simulink model "simulation2_Fault"  (R2018a)
settings: Solver=FixedStepAuto  StartTime=0.0  StopTime=2000  FixedStep=0.1  RelTol=1e-3
values from neighbouring files (symbols this model uses):
  C_wn = C_w(:,4)    [Sim1.m]    (also in Sim3.m; Sim4_EKF.m; Sim4_Nolinear.m; Sim5_Nolinear.m)
  C_wx = C_w(:,2)    [Sim1.m]    (also in Sim3.m; Sim4_EKF.m; Sim4_Nolinear.m; Sim5_Nolinear.m)
  C_wy = C_w(:,3)    [Sim1.m]    (also in Sim3.m; Sim4_EKF.m; Sim4_Nolinear.m; Sim5_Nolinear.m)
  Ce = inv(W)*Be'/(Be/W*Be')    [Sim2.m]    (also in Sim3.m; Sim4_EKF.m; Sim4_Nolinear.m; Sim5_Nolinear.m)
  getPos = [0;0;1]    [Sim2.m]    (also in Sim3.m; Sim4_EKF.m; Sim4_Nolinear.m; Sim5_Nolinear.m)
  getVel = [0;1;0]    [Sim2.m]    (also in Sim3.m; Sim4_EKF.m; Sim4_Nolinear.m; Sim5_Nolinear.m)
  h = 0.1    [Sim1.m]    (also in Sim2.m; Sim3.m; Sim4_EKF.m; Sim4_Nolinear.m)
  Kd = 7*[2*M3(1)*Omega 0 0; 0 3*M3(2,2)*Omega 0; 0 0 20*M(3,3)*Omega]    [Sim2.m]    (also in Sim3.m; Sim4_EKF.m; Sim4_Nolinear.m; Sim5_Nolinear.m = 7*[30*M3(1)*Omega 0 0; 0 150*M3(2,2)*Omega 0; 0 0 30*M(3,3)*)
  Ki = 100*(omega/10)*[M3(1)*omega^2 0 0;0 0.05*M3(2,2)*omega^2 0; 0 0 M3(3,3)*omega^2 ]*2    [Sim2.m]    (also in Sim3.m; Sim4_EKF.m; Sim4_Nolinear.m; Sim5_Nolinear.m = 10*(omega/10)*[30*M3(1)*omega^2 0 0;0 150*M3(2,2)*omega^2 0;)
  Kp = 50*[6*M3(1)*omega^2 0 0;0 M3(2,2)*omega^2 0; 0 0 10*M3(3,3)*omega^2 ]    [Sim2.m]    (also in Sim3.m; Sim4_EKF.m; Sim4_Nolinear.m; Sim5_Nolinear.m = 5*[60*M3(1)*omega^2 0 0;0 800*M3(2,2)*omega^2 0; 0 0 30*M3(3)
  mu2_c = 0.001    [Sim1.m]    (also in Sim3.m; Sim4_EKF.m; Sim4_Nolinear.m; Sim5_Nolinear.m)
  mu2_w = 0.001    [Sim1.m]    (also in Sim3.m; Sim4_EKF.m; Sim4_Nolinear.m; Sim5_Nolinear.m)
  mu_w = 0.001    [Sim1.m]    (also in Sim3.m; Sim4_EKF.m; Sim4_Nolinear.m; Sim5_Nolinear.m)
  Omega = 2*damping*omega    [Sim2.m]    (also in Sim3.m; Sim4_EKF.m; Sim4_Nolinear.m = diag([omega_1,omega_2,omega_3]); Sim5_Nolinear.m = diag([omega_1,omega_2,omega_3]))
  omega = omegab/sqrt(1-2*damping^2+sqrt(4*damping^4-4*damping^2+2))    [Sim2.m]    (also in Sim3.m; Sim4_EKF.m; Sim4_Nolinear.m; Sim5_Nolinear.m)
  phi_c = -pi/2    (= -1.57079632679)    [Sim1.m]    (also in Sim3.m; Sim4_EKF.m; Sim4_Nolinear.m; Sim5_Nolinear.m)
  psi_r = C_w(:,1)    [Sim1.m]    (also in Sim3.m; Sim4_EKF.m; Sim4_Nolinear.m; Sim5_Nolinear.m)
  rotationspeed_3 = 4*pi    (= 12.5663706144)    [Sim2.m]    (also in Sim3.m; Sim4_EKF.m; Sim4_Nolinear.m; Sim5_Nolinear.m)
  rotationspeed_5 = 4*pi    (= 12.5663706144)    [Sim2.m]    (also in Sim3.m; Sim4_EKF.m; Sim4_Nolinear.m; Sim5_Nolinear.m)
  rotationspeed_6 = 4*pi    (= 12.5663706144)    [Sim2.m]    (also in Sim3.m; Sim4_EKF.m; Sim4_Nolinear.m; Sim5_Nolinear.m)
  thrust_1 = 420000    [Sim2.m]    (also in Sim3.m; Sim4_EKF.m; Sim4_Nolinear.m; Sim5_Nolinear.m)
  thrust_2 = 420000    [Sim2.m]    (also in Sim3.m; Sim4_EKF.m; Sim4_Nolinear.m; Sim5_Nolinear.m)
  thrust_3 = 500000    [Sim2.m]    (also in Sim3.m; Sim4_EKF.m; Sim4_Nolinear.m; Sim5_Nolinear.m)
  thrust_4 = 260000    [Sim2.m]    (also in Sim3.m; Sim4_EKF.m; Sim4_Nolinear.m; Sim5_Nolinear.m)
  thrust_5 = 1100000    [Sim2.m]    (also in Sim3.m; Sim4_EKF.m; Sim4_Nolinear.m; Sim5_Nolinear.m)
  thrust_6 = 1100000    [Sim2.m]    (also in Sim3.m; Sim4_EKF.m; Sim4_Nolinear.m; Sim5_Nolinear.m)
  thrustrate_1 = 420000/8    (= 52500)    [Sim2.m]    (also in Sim3.m; Sim4_EKF.m; Sim4_Nolinear.m; Sim5_Nolinear.m)
  thrustrate_2 = 420000/8    (= 52500)    [Sim2.m]    (also in Sim3.m; Sim4_EKF.m; Sim4_Nolinear.m; Sim5_Nolinear.m)
  thrustrate_3 = 500000/8    (= 62500)    [Sim2.m]    (also in Sim3.m; Sim4_EKF.m; Sim4_Nolinear.m; Sim5_Nolinear.m)
  thrustrate_4 = 260000/8    (= 32500)    [Sim2.m]    (also in Sim3.m; Sim4_EKF.m; Sim4_Nolinear.m; Sim5_Nolinear.m)
  thrustrate_5 = 1100000/12    (= 91666.6666667)    [Sim2.m]    (also in Sim3.m; Sim4_EKF.m; Sim4_Nolinear.m; Sim5_Nolinear.m)
  thrustrate_6 = 1100000/12    (= 91666.6666667)    [Sim2.m]    (also in Sim3.m; Sim4_EKF.m; Sim4_Nolinear.m; Sim5_Nolinear.m)
  V_mean = 0.5    [Sim1.m]    (also in Sim3.m; Sim4_EKF.m; Sim4_Nolinear.m; Sim5_Nolinear.m)
  W_gust = Ug    [Sim1.m]    (also in Sim3.m; Sim4_EKF.m; Sim4_Nolinear.m; Sim5_Nolinear.m)
  W_mean = 15    [Sim1.m]    (also in Sim3.m; Sim4_EKF.m; Sim4_Nolinear.m; Sim5_Nolinear.m)
  xposition = [77, 74, 70, -65, -72, -72]    [Sim2.m]    (also in Sim3.m; Sim4_EKF.m; Sim4_Nolinear.m; Sim5_Nolinear.m)
  yposition = [0, 0, 0, 0, 5, -5]    [Sim2.m]    (also in Sim3.m; Sim4_EKF.m; Sim4_Nolinear.m; Sim5_Nolinear.m)
undefined symbols (not defined in the file or in its folder): Hoerner, magnitude, sigbuilder_block, vessel
libraries: simulink x3, marine_hydro x2, marine_gnc x1, simulink_extras x1
settings Model: Creator=jonbjor  LastModifiedBy=34275

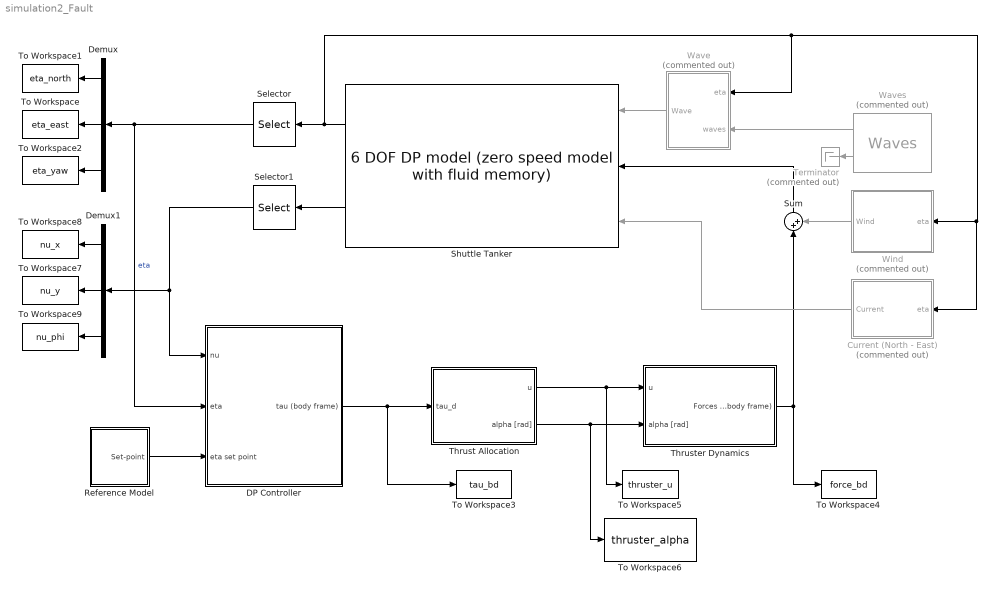
== system simulation2_Fault ==
  Current (North - East) : Subsystem  Commented=on
  DP Controller : Subsystem
  Demux : Demux  Outputs=3
  Demux1 : Demux  Outputs=3
  Reference Model : Subsystem
  Selector : Selector  InputPortWidth=6  IndexOptions=Index vector (dialog)  Indices=[1 2 6]  OutputSizes=1
  Selector1 : Selector  InputPortWidth=6  IndexOptions=Index vector (dialog)  Indices=[1 2 6]  OutputSizes=1
  Shuttle Tanker : marine_hydro/Hydro Library/6 DOF DP model  (zero speed model with fluid memory)  ABC=vesselABC  rho=1025  Axc=0.9*vessel.main.T*vessel.main.B  Ayc=0.9*vessel.main.T*vessel.main.Lpp  CX=1  CY_2D=Hoerner(vessel.main.B,vessel.main.T)  Bv=vessel.Bv  mask(6 DOF zero speed model){}
      link override "Integrator1 ": InitialCondition=nu0
      link override Integrator2: InitialCondition=eta0
      settings: SourceProductName=MSS Hydro
      mask Display:
      | image('shuttleTanker.jpg');
      | color('white'); port_label('output', 1, 'eta')
      | color('white'); port_label('output', 2, 'nu')
      | color('white'); port_label('input', 1, 'tau_wave')
      | color('white'); port_label('input', 2, 'tau')
      | color('white'); port_label('input', 3, 'nu_c')
  Sum : Sum  Inputs=|++
  Terminator : Terminator  Commented=on
  Thrust Allocation : Subsystem
  Thruster Dynamics : Subsystem  mask{thrusterfault=on}
      mask prompts: thrusterfault "Fault on thruster #2 and #5?"
  To Workspace : ToWorkspace  VariableName=eta_east  SaveFormat=Timeseries  SampleTime=-1
  To Workspace1 : ToWorkspace  VariableName=eta_north  SaveFormat=Timeseries  SampleTime=-1
  To Workspace2 : ToWorkspace  VariableName=eta_yaw  SaveFormat=Timeseries  SampleTime=-1
  To Workspace3 : ToWorkspace  VariableName=tau_bd  SaveFormat=Timeseries  SampleTime=-1
  To Workspace4 : ToWorkspace  VariableName=force_bd  SaveFormat=Timeseries  SampleTime=-1
  To Workspace5 : ToWorkspace  VariableName=thruster_u  SaveFormat=Timeseries  SampleTime=-1
  To Workspace6 : ToWorkspace  VariableName=thruster_alpha  SaveFormat=Timeseries  SampleTime=-1
  To Workspace7 : ToWorkspace  VariableName=nu_y  SaveFormat=Timeseries  SampleTime=-1
  To Workspace8 : ToWorkspace  VariableName=nu_x  SaveFormat=Timeseries  SampleTime=-1
  To Workspace9 : ToWorkspace  VariableName=nu_phi  SaveFormat=Timeseries  SampleTime=-1
  Wave : Subsystem  Commented=on  mask{waveforces=on}
      mask prompts: waveforces "Waveforces enabled"
  Waves : marine_gnc/Environment/Waves/Waves  Commented=on  spectrum_type=ITTC  disp_flag=on  plot_spectrum=off  plot_realization=off  hs=5  omega_peak=pi/10  psi_mean=0  gamma=-1  spread=2  depth=inf  nfreq=20  ndir=10  energylim=0.005  freq_cutoff=3  dir_cutoff=0  rand_seed=123  rand_freq=on  rand_dir=on  Zeta_a=0  Omega=0  Phase=0  Wavenum=0  Psi=0
      settings: SourceProductName=MSS GNC
  Wind : Subsystem  Commented=on
  wires:
  Shuttle Tanker/2 -> Selector1/1
  Reference Model/1(Set-point) -> DP Controller/3(eta set point)
  DP Controller/1(tau (body frame)) -> To Workspace3/1, Thrust Allocation/1(tau_d)
  Shuttle Tanker/1 -> Selector/1, Current (North - East)/1(eta), Wind/1(eta), Wave/1(eta)
  Wave/1(Wave) -> Shuttle Tanker/1
  Waves/1 -> Wave/2(waves)
  Waves/2 -> Terminator/1
  Selector1/1 -> DP Controller/1(nu), Demux1/1
  Thrust Allocation/1(u) -> To Workspace5/1, Thruster Dynamics/1(u)
  Wind/1(Wind) -> Sum/2
  Thruster Dynamics/1("Forces (body frame) ") -> To Workspace4/1, Sum/1
  Sum/1 -> Shuttle Tanker/2
  Thrust Allocation/2(alpha [rad]) -> To Workspace6/1, Thruster Dynamics/2(alpha [rad])
  Selector/1 -> DP Controller/2(eta), Demux/1  "eta"
  Demux/3 -> To Workspace2/1
  Current (North - East)/1(Current) -> Shuttle Tanker/3
  Demux/1 -> To Workspace1/1
  Demux/2 -> To Workspace/1
  Demux1/3 -> To Workspace9/1
  Demux1/1 -> To Workspace8/1
  Demux1/2 -> To Workspace7/1

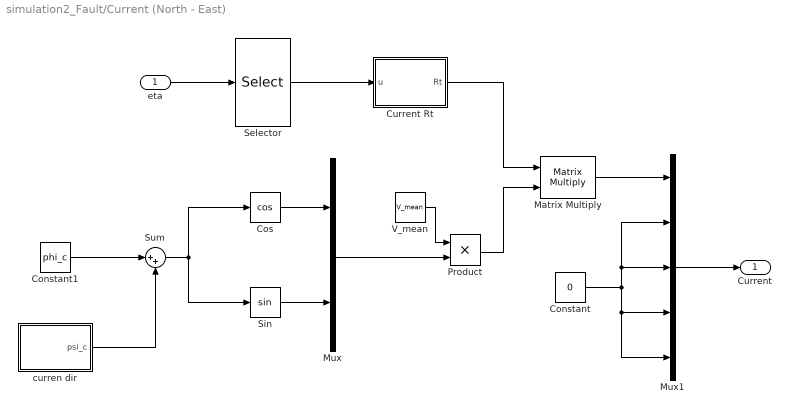
== system simulation2_Fault/Current (North - East) ==
  eta : Inport
  Constant : Constant  Value=0
  Constant1 : Constant  Value=phi_c
  Cos : Trigonometry  Operator=cos
  Current Rt : MATLAB Function  TreatAsAtomicUnit=on
  Matrix Multiply : Product  Multiplication=Matrix(*)
  Mux : Mux  Inputs=2
  Mux1 : Mux  Inputs=5
  Product : Product
  Selector : Selector  InputPortWidth=6  IndexOptions=Index vector (dialog)  Indices=[6]  OutputSizes=1
  Sin : Trigonometry
  Sum : Sum  Inputs=|++
  V_mean : Constant  Value=V_mean
  curren dir : Subsystem
  Current : Outport
  wires:
  V_mean/1 -> Product/1
  Mux1/1 -> Current/1
  Cos/1 -> Mux/1
  Mux/1 -> Product/2
  Sin/1 -> Mux/2
  Constant/1 -> Mux1/5, Mux1/4, Mux1/3, Mux1/2
  Constant1/1 -> Sum/1
  curren dir/1("psi_c ") -> Sum/2
  Sum/1 -> Sin/1, Cos/1
  eta/1 -> Selector/1
  Selector/1 -> Current Rt/1(u)
  Current Rt/1(Rt) -> Matrix Multiply/1
  Product/1 -> Matrix Multiply/2
  Matrix Multiply/1 -> Mux1/1

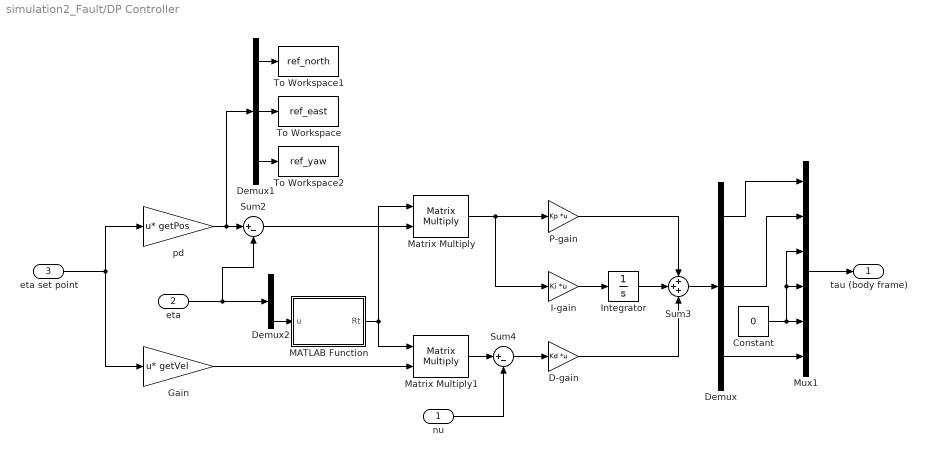
== system simulation2_Fault/DP Controller ==
  nu : Inport
  eta : Inport  Port=2
  eta set point : Inport  Port=3
  Constant : Constant  Value=0
  D-gain : Gain  Gain=Kd  Multiplication=Matrix(K*u)
  Demux : Demux  Outputs=3
  Demux1 : Demux  Outputs=3
  Demux2 : Demux  Outputs=3
  Gain : Gain  Gain=getVel  Multiplication=Matrix(u*K)
  I-gain : Gain  Gain=Ki  Multiplication=Matrix(K*u)
  Integrator : Integrator
  MATLAB Function : MATLAB Function  TreatAsAtomicUnit=on
  Matrix Multiply : Product  Multiplication=Matrix(*)
  Matrix Multiply1 : Product  Multiplication=Matrix(*)
  Mux1 : Mux  Inputs=6
  P-gain : Gain  Gain=Kp  Multiplication=Matrix(K*u)
  Sum2 : Sum  Inputs=|+-
  Sum3 : Sum  Inputs=+++
  Sum4 : Sum  Inputs=|+-
  To Workspace : ToWorkspace  VariableName=ref_east  SaveFormat=Timeseries  SampleTime=-1
  To Workspace1 : ToWorkspace  VariableName=ref_north  SaveFormat=Timeseries  SampleTime=-1
  To Workspace2 : ToWorkspace  VariableName=ref_yaw  SaveFormat=Timeseries  SampleTime=-1
  pd : Gain  Gain=getPos  Multiplication=Matrix(u*K)
  tau (body frame) : Outport
  wires:
  Demux2/3 -> MATLAB Function/1(u)
  pd/1 -> Demux1/1, Sum2/1
  Matrix Multiply/1 -> I-gain/1, P-gain/1
  Mux1/1 -> tau (body frame)/1
  Demux/3 -> Mux1/6
  Integrator/1 -> Sum3/2
  Demux/2 -> Mux1/2
  P-gain/1 -> Sum3/1
  nu/1 -> Sum4/2
  Sum2/1 -> Matrix Multiply/2
  D-gain/1 -> Sum3/3
  MATLAB Function/1(Rt) -> Matrix Multiply1/1, Matrix Multiply/1
  Demux/1 -> Mux1/1
  Matrix Multiply1/1 -> Sum4/1
  Constant/1 -> Mux1/4, Mux1/3, Mux1/5
  eta set point/1 -> Gain/1, pd/1
  Gain/1 -> Matrix Multiply1/2
  Sum3/1 -> Demux/1
  Sum4/1 -> D-gain/1
  I-gain/1 -> Integrator/1
  eta/1 -> Demux2/1, Sum2/2
  Demux1/1 -> To Workspace1/1
  Demux1/3 -> To Workspace2/1
  Demux1/2 -> To Workspace/1

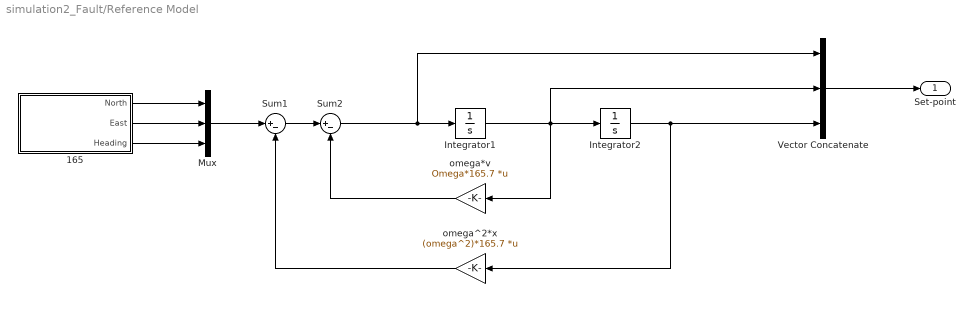
== system simulation2_Fault/Reference Model ==
  165 : Subsystem  Tag=STV Subsys  LoadFcn=sigbuilder_block('load');  StartFcn=sigbuilder_block('start');  StopFcn=sigbuilder_block('stop');  ClipboardFcn=sigbuilder_block('clipboard');  mask(Sigbuilder block){tuvar=[0:10]}
      mask help: Simulink:masks:SigbuilderBlock_MD
      mask init:
      | if ~strcmp(get_param(bdroot(gcbh),'SimulationStatus'),'stopped') tuvar = sigbuilder_block('maskInit'); end
      settings: CopyFcn=sigbuilder_block('copy');  DeleteFcn=sigbuilder_block('delete');  ModelCloseFcn=sigbuilder_block('modelClose');  PreSaveFcn=sigbuilder_block('preSave');  PauseFcn=sigbuilder_block('pause');  ContinueFcn=sigbuilder_block('continue');  NameChangeFcn=sigbuilder_block('namechange');  OpenFcn=sigbuilder_block('open',[5.4 30 1141.2 523.8 ]);  CloseFcn=sigbuilder_block('close');
      mask Display: plot(0, 0, 100, 100,[2, 2, 32, 32, 2], [68, 8, 8, 68, 68],[32, 2], [38, 38], [32, 19, 2],[53, 60, 44], [32, 17, 17, 2],[16, 16, 31, 31]);txt = getActiveGroup(gcbh);text(2, 100, txt,'verticalAlignment', 'top');
  Integrator1 : Integrator
  Integrator2 : Integrator
  Mux : Mux  Inputs=3
  Sum1 : Sum  Inputs=|+-
  Sum2 : Sum  Inputs=|+-
  Vector Concatenate : Concatenate  NumInputs=3  Mode=Multidimensional array  ConcatenateDimension=2
  omega*v : Gain  Gain=Omega*165.7  Multiplication=Matrix(K*u)
  omega^2*x : Gain  Gain=(omega^2)*165.7  Multiplication=Matrix(K*u)
  Set-point : Outport
  wires:
  omega*v/1 -> Sum2/2
  Sum1/1 -> Sum2/1
  omega^2*x/1 -> Sum1/2
  Sum2/1 -> Vector Concatenate/1, Integrator1/1
  Integrator2/1 -> omega^2*x/1, Vector Concatenate/3
  Integrator1/1 -> omega*v/1, Vector Concatenate/2, Integrator2/1
  Vector Concatenate/1 -> Set-point/1
  165/1(North) -> Mux/1
  165/2(East) -> Mux/2
  165/3(Heading) -> Mux/3
  Mux/1 -> Sum1/1

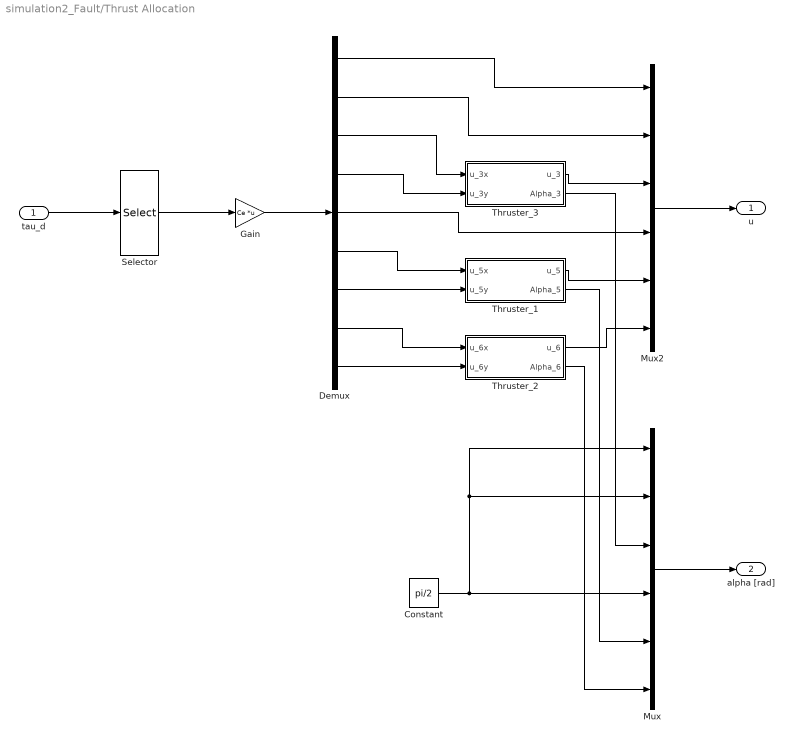
== system simulation2_Fault/Thrust Allocation ==
  tau_d : Inport
  Constant : Constant  Value=pi/2
  Demux : Demux  Outputs=9
  Gain : Gain  Gain=Ce  Multiplication=Matrix(K*u)
  Mux : Mux  Inputs=6
  Mux2 : Mux  Inputs=6
  Selector : Selector  InputPortWidth=6  IndexOptions=Index vector (dialog)  Indices=[1 2 6]  OutputSizes=1
  Thruster_1 : Subsystem
  Thruster_2 : Subsystem
  Thruster_3 : Subsystem
  u : Outport
  alpha [rad] : Outport  Port=2
  wires:
  tau_d/1 -> Selector/1
  Constant/1 -> Mux/4, Mux/2, Mux/1
  Mux/1 -> alpha [rad]/1
  Gain/1 -> Demux/1
  Mux2/1 -> u/1
  Demux/1 -> Mux2/1
  Demux/2 -> Mux2/2
  Demux/5 -> Mux2/4
  Demux/3 -> Thruster_3/1(u_3x)
  Demux/4 -> Thruster_3/2(u_3y)
  Thruster_3/1(u_3) -> Mux2/3
  Thruster_1/1(u_5) -> Mux2/5
  Thruster_2/1(u_6) -> Mux2/6
  Demux/6 -> Thruster_1/1(u_5x)
  Demux/7 -> Thruster_1/2(u_5y)
  Demux/8 -> Thruster_2/1(u_6x)
  Demux/9 -> Thruster_2/2(u_6y)
  Thruster_3/2(Alpha_3) -> Mux/3
  Thruster_1/2(Alpha_5) -> Mux/5
  Thruster_2/2(Alpha_6) -> Mux/6
  Selector/1 -> Gain/1

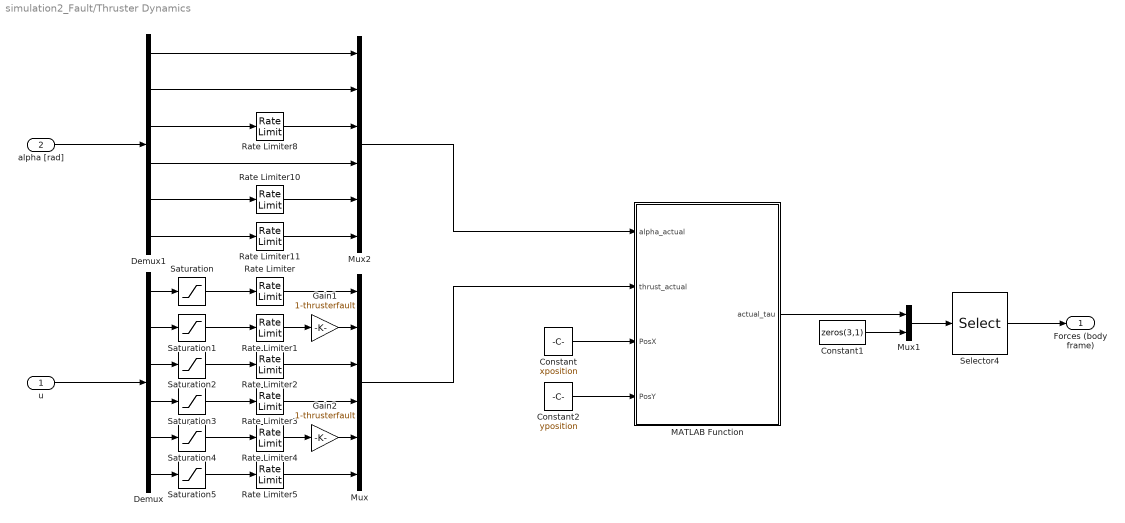
== system simulation2_Fault/Thruster Dynamics ==
  u : Inport
  alpha [rad] : Inport  Port=2
  Constant : Constant  Value=xposition
  Constant1 : Constant  Value=zeros(3,1)
  Constant2 : Constant  Value=yposition
  Demux : Demux  Outputs=6
  Demux1 : Demux  Outputs=6
  Gain1 : Gain  Gain=1-thrusterfault
  Gain2 : Gain  Gain=1-thrusterfault
  MATLAB Function : MATLAB Function  TreatAsAtomicUnit=on
  Mux : Mux  Inputs=6
  Mux1 : Mux  Inputs=2
  Mux2 : Mux  Inputs=6
  Rate Limiter : RateLimiter  RisingSlewLimit=thrustrate_1  FallingSlewLimit=-thrustrate_1  SampleTimeMode=inherited
  Rate Limiter1 : RateLimiter  RisingSlewLimit=thrustrate_2  FallingSlewLimit=-thrustrate_2  SampleTimeMode=inherited
  Rate Limiter10 : RateLimiter  RisingSlewLimit=rotationspeed_5  FallingSlewLimit=-rotationspeed_5  SampleTimeMode=inherited
  Rate Limiter11 : RateLimiter  RisingSlewLimit=rotationspeed_6  FallingSlewLimit=-rotationspeed_6  SampleTimeMode=inherited
  Rate Limiter2 : RateLimiter  RisingSlewLimit=thrustrate_3  FallingSlewLimit=-thrustrate_3  SampleTimeMode=inherited
  Rate Limiter3 : RateLimiter  RisingSlewLimit=thrustrate_4  FallingSlewLimit=-thrustrate_4  SampleTimeMode=inherited
  Rate Limiter4 : RateLimiter  RisingSlewLimit=thrustrate_5  FallingSlewLimit=-thrustrate_5  SampleTimeMode=inherited
  Rate Limiter5 : RateLimiter  RisingSlewLimit=thrustrate_6  FallingSlewLimit=-thrustrate_6  SampleTimeMode=inherited
  Rate Limiter8 : RateLimiter  RisingSlewLimit=rotationspeed_3  FallingSlewLimit=-rotationspeed_3  SampleTimeMode=inherited
  Saturation : Saturate  UpperLimit=thrust_1  LowerLimit=-thrust_1
  Saturation1 : Saturate  UpperLimit=thrust_2  LowerLimit=-thrust_2
  Saturation2 : Saturate  UpperLimit=thrust_3  LowerLimit=-thrust_3
  Saturation3 : Saturate  UpperLimit=thrust_4  LowerLimit=-thrust_4
  Saturation4 : Saturate  UpperLimit=thrust_5  LowerLimit=-thrust_5
  Saturation5 : Saturate  UpperLimit=thrust_6  LowerLimit=-thrust_6
  Selector4 : Selector  InputPortWidth=6  IndexOptions=Index vector (dialog)  Indices=[1 2 4 5 6 3]  OutputSizes=1
  "Forces (body frame) " : Outport
  wires:
  Rate Limiter2/1 -> Mux/3
  Saturation/1 -> Rate Limiter/1
  Mux1/1 -> Selector4/1
  Constant1/1 -> Mux1/2
  Demux/5 -> Saturation4/1
  Demux/4 -> Saturation3/1
  Saturation4/1 -> Rate Limiter4/1
  Demux/2 -> Saturation1/1
  Saturation1/1 -> Rate Limiter1/1
  Demux/1 -> Saturation/1
  Demux/3 -> Saturation2/1
  Saturation2/1 -> Rate Limiter2/1
  Saturation3/1 -> Rate Limiter3/1
  Selector4/1 -> "Forces (body frame) "/1
  Gain1/1 -> Mux/2
  Rate Limiter3/1 -> Mux/4
  Rate Limiter1/1 -> Gain1/1
  Rate Limiter/1 -> Mux/1
  Rate Limiter4/1 -> Gain2/1
  Saturation5/1 -> Rate Limiter5/1
  Demux/6 -> Saturation5/1
  Rate Limiter5/1 -> Mux/6
  Gain2/1 -> Mux/5
  Demux1/6 -> Rate Limiter11/1
  Demux1/3 -> Rate Limiter8/1
  Rate Limiter11/1 -> Mux2/6
  Rate Limiter10/1 -> Mux2/5
  Demux1/2 -> Mux2/2
  Demux1/1 -> Mux2/1
  Demux1/4 -> Mux2/4
  Rate Limiter8/1 -> Mux2/3
  Demux1/5 -> Rate Limiter10/1
  u/1 -> Demux/1
  alpha [rad]/1 -> Demux1/1
  Constant/1 -> MATLAB Function/3(PosX)
  Constant2/1 -> MATLAB Function/4(PosY)
  Mux/1 -> MATLAB Function/2(thrust_actual)
  Mux2/1 -> MATLAB Function/1(alpha_actual)
  MATLAB Function/1(actual_tau) -> Mux1/1

== system simulation2_Fault/Wave ==
  eta : Inport
  waves : Inport  Port=2
  Gain : Gain  Gain=waveforces
  Sum : Sum
  Wave loads (U=0) : marine_hydro/Hydro Library/Wave loads (U=0)
      settings: SourceProductName=MSS Hydro
  Wave : Outport
  wires:
  eta/1 -> Wave loads (U=0)/1
  waves/1 -> Wave loads (U=0)/2
  Sum/1 -> Gain/1
  Wave loads (U=0)/1 -> Sum/1
  Wave loads (U=0)/2 -> Sum/2
  Gain/1 -> Wave/1

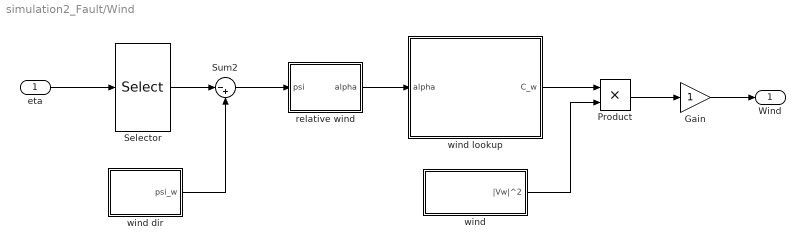
== system simulation2_Fault/Wind ==
  eta : Inport
  Gain : Gain
  Product : Product
  Selector : Selector  InputPortWidth=6  IndexOptions=Index vector (dialog)  Indices=[6]  OutputSizes=1
  Sum2 : Sum  Inputs=|-+
  relative wind : MATLAB Function  TreatAsAtomicUnit=on
  wind : Subsystem
  wind dir : Subsystem
  wind lookup : Subsystem
  Wind : Outport
  wires:
  wind lookup/1(C_w) -> Product/1
  relative wind/1(alpha) -> wind lookup/1(alpha)
  Sum2/1 -> relative wind/1(psi)
  wind dir/1(psi_w) -> Sum2/2
  wind/1(|Vw|^2) -> Product/2
  Product/1 -> Gain/1
  eta/1 -> Selector/1
  Selector/1 -> Sum2/1
  Gain/1 -> Wind/1

== system simulation2_Fault/Current (North - East)/curren dir ==
  Add : Sum  Inputs=+-
  Band-Limited White Noise : simulink/Sources/Band-Limited White Noise  Cov=w  Ts=h  seed=[23341]
  Constant : Constant  Value=mu2_c
  Integrator : Integrator
  Saturation : Saturate  UpperLimit=5*pi/180  LowerLimit=5*pi/180
  prod : Product  Inputs=**
  "psi_c " : Outport
  wires:
  Add/1 -> Integrator/1  "psidot"
  prod/1 -> Add/2
  Band-Limited White Noise/1 -> Add/1
  Constant/1 -> prod/1
  Integrator/1 -> Saturation/1, prod/2
  Saturation/1 -> "psi_c "/1

== system simulation2_Fault/Reference Model/165 ==
  Demux : Demux  Tag=STV Demux  Outputs=3
  FromWs : FromWorkspace  Tag=STV FromWs  VariableName=tuvar  SampleTime=0
      SigBuilderData=|
      | common.afterFinalStr = 'Extrapolate'
      | common.sampleTime = 0
      | dataSet.timeRange = [0 2000]
      | dataSet.name = 'Group 1'
      | sbobj.Groups.Name = 'Group 1'
      | sbobj.Groups.Signals(1).Name = 'North'
      | sbobj.Groups.Signals(1).XData = [0 165 850 1100 2000]
      | sbobj.Groups.Signals(1).YData = [0 50 50 0 0]
      | sbobj.Groups.Signals(2).Name = 'East'
      | sbobj.Groups.Signals(2).XData = [0 400 565 1400 1565 2000]
      | sbobj.Groups.Signals(2).YData = [0 0 -50 -50 0 0]
      | sbobj.Groups.Signals(3).Name = 'Heading'
      | sbobj.Groups.Signals(3).XData = [0 850 1100 2000]
      | sbobj.Groups.Signals(3).YData = [0 0 -1.57079632679 -1.57079632679]
      | sbobj.Groups.TimeRange = [0 2000]
  North : Outport  Tag=STV Outport
  East : Outport  Tag=STV Outport  Port=2
  Heading : Outport  Tag=STV Outport  Port=3
  wires:
  FromWs/1 -> Demux/1
  Demux/1 -> North/1
  Demux/2 -> East/1
  Demux/3 -> Heading/1

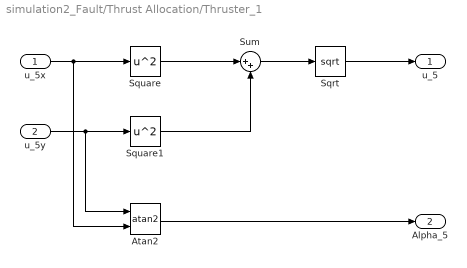
== system simulation2_Fault/Thrust Allocation/Thruster_1 ==
  u_5x : Inport
  u_5y : Inport  Port=2
  Atan2 : Trigonometry  Operator=atan2
  Sqrt : Sqrt  SaturateOnIntegerOverflow=on
  Square : Math  Operator=square  SaturateOnIntegerOverflow=on
  Square1 : Math  Operator=square  SaturateOnIntegerOverflow=on
  Sum : Sum  Inputs=|++
  u_5 : Outport
  Alpha_5 : Outport  Port=2
  wires:
  Square/1 -> Sum/1
  Square1/1 -> Sum/2
  Sum/1 -> Sqrt/1
  Sqrt/1 -> u_5/1
  u_5x/1 -> Atan2/2, Square/1
  Atan2/1 -> Alpha_5/1
  u_5y/1 -> Atan2/1, Square1/1

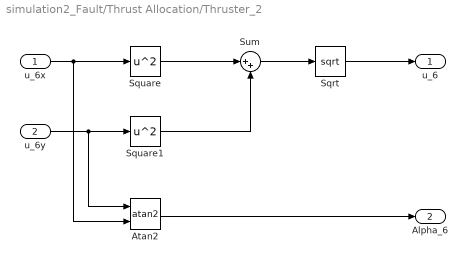
== system simulation2_Fault/Thrust Allocation/Thruster_2 ==
  u_6x : Inport
  u_6y : Inport  Port=2
  Atan2 : Trigonometry  Operator=atan2
  Sqrt : Sqrt  SaturateOnIntegerOverflow=on
  Square : Math  Operator=square  SaturateOnIntegerOverflow=on
  Square1 : Math  Operator=square  SaturateOnIntegerOverflow=on
  Sum : Sum  Inputs=|++
  u_6 : Outport
  Alpha_6 : Outport  Port=2
  wires:
  Square/1 -> Sum/1
  Square1/1 -> Sum/2
  Sum/1 -> Sqrt/1
  Sqrt/1 -> u_6/1
  u_6x/1 -> Atan2/2, Square/1
  Atan2/1 -> Alpha_6/1
  u_6y/1 -> Atan2/1, Square1/1

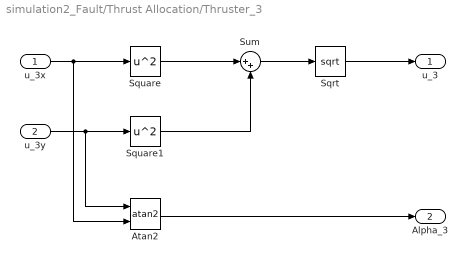
== system simulation2_Fault/Thrust Allocation/Thruster_3 ==
  u_3x : Inport
  u_3y : Inport  Port=2
  Atan2 : Trigonometry  Operator=atan2
  Sqrt : Sqrt  SaturateOnIntegerOverflow=on
  Square : Math  Operator=square  SaturateOnIntegerOverflow=on
  Square1 : Math  Operator=square  SaturateOnIntegerOverflow=on
  Sum : Sum  Inputs=|++
  u_3 : Outport
  Alpha_3 : Outport  Port=2
  wires:
  u_3x/1 -> Atan2/2, Square/1
  u_3y/1 -> Square1/1, Atan2/1
  Square/1 -> Sum/1
  Square1/1 -> Sum/2
  Sum/1 -> Sqrt/1
  Sqrt/1 -> u_3/1
  Atan2/1 -> Alpha_3/1

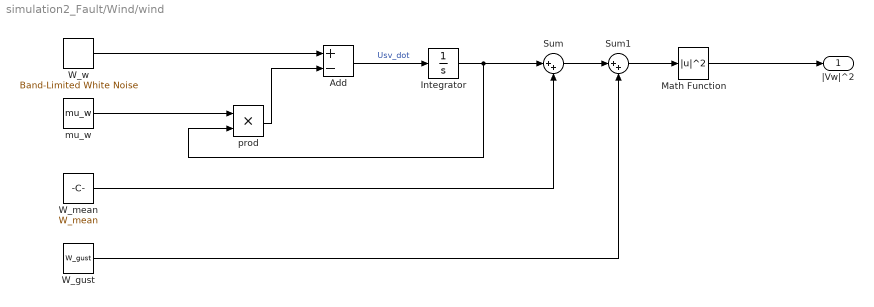
== system simulation2_Fault/Wind/wind ==
  Add : Sum  Inputs=+-
  Integrator : Integrator
  Math Function : Math  Operator=magnitude^2  SaturateOnIntegerOverflow=on
  Sum : Sum  Inputs=|++
  Sum1 : Sum  Inputs=|++
  W_gust : Constant  Value=W_gust
  "W_mean " : Constant  Value=W_mean
  W_w : simulink/Sources/Band-Limited White Noise  Cov=w  Ts=0.1  seed=[23341]
  mu_w : Constant  Value=mu_w
  prod : Product  Inputs=**
  |Vw|^2 : Outport
  wires:
  Add/1 -> Integrator/1  "Usv_dot"
  prod/1 -> Add/2
  Math Function/1 -> |Vw|^2/1
  "W_mean "/1 -> Sum/2
  W_w/1 -> Add/1
  mu_w/1 -> prod/1
  Integrator/1 -> Sum/1, prod/2
  W_gust/1 -> Sum1/2
  Sum/1 -> Sum1/1
  Sum1/1 -> Math Function/1

== system simulation2_Fault/Wind/wind dir ==
  Add : Sum  Inputs=+-
  Band-Limited White Noise : simulink/Sources/Band-Limited White Noise  Cov=w  Ts=h  seed=[23341]
  Constant : Constant  Value=mu2_w
  Integrator : Integrator
  Saturation : Saturate  UpperLimit=5*pi/180  LowerLimit=5*pi/180
  prod : Product  Inputs=**
  psi_w : Outport
  wires:
  Add/1 -> Integrator/1  "psidot"
  prod/1 -> Add/2
  Band-Limited White Noise/1 -> Add/1
  Constant/1 -> prod/1
  Integrator/1 -> Saturation/1, prod/2
  Saturation/1 -> psi_w/1

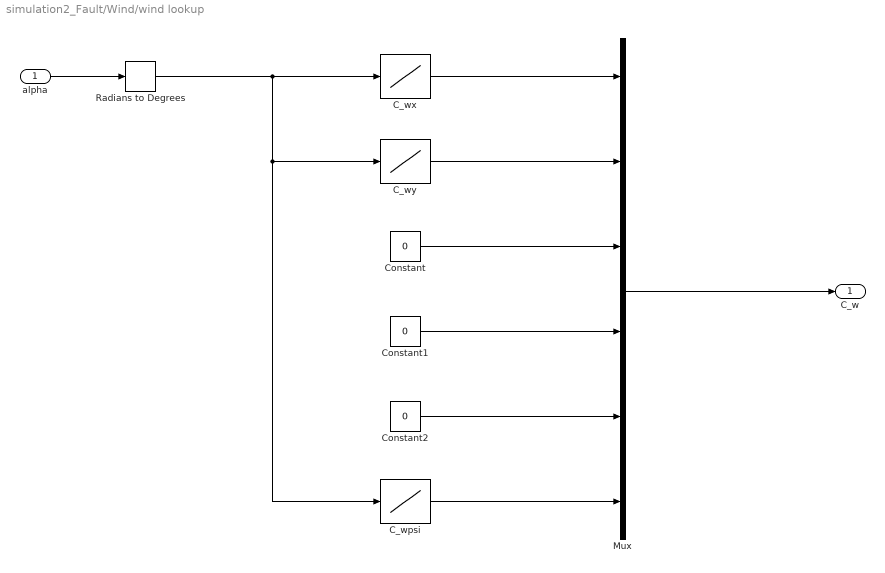
== system simulation2_Fault/Wind/wind lookup ==
  alpha : Inport
  C_wpsi : Lookup_n-D  NumberOfTableDimensions=1  BreakpointsForDimension1=psi_r  Table=C_wn  InternalRulePriority=Speed  RndMeth=Simplest  InputSameDT=on
  C_wx : Lookup_n-D  NumberOfTableDimensions=1  BreakpointsForDimension1=psi_r  Table=C_wx  InternalRulePriority=Speed  RndMeth=Simplest  InputSameDT=on
  C_wy : Lookup_n-D  NumberOfTableDimensions=1  BreakpointsForDimension1=psi_r  Table=C_wy  InternalRulePriority=Speed  RndMeth=Simplest  InputSameDT=on
  Constant : Constant  Value=0
  Constant1 : Constant  Value=0
  Constant2 : Constant  Value=0
  Mux : Mux  Inputs=6
  Radians to Degrees : simulink_extras/Transformations/Radians to Degrees
  C_w : Outport
  wires:
  C_wx/1 -> Mux/1
  C_wy/1 -> Mux/2
  Constant/1 -> Mux/3
  Constant1/1 -> Mux/4
  Constant2/1 -> Mux/5
  C_wpsi/1 -> Mux/6
  Mux/1 -> C_w/1
  alpha/1 -> Radians to Degrees/1
  Radians to Degrees/1 -> C_wpsi/1, C_wy/1, C_wx/1

== matlab function simulation2_Fault/DP Controller/MATLAB Function ==
  data: u input; Rt output
function Rt = fcn(u)

R=[cos(u) -sin(u) 0; sin(u) cos(u) 0; 0 0 1];
Rt=transpose(R);

end

== matlab function simulation2_Fault/Wind/relative wind ==
  data: psi input; alpha output
function alpha = psi2alpha(psi)

alph = pi-psi;

if alph < 0
    alph = alph+2*pi;
end

alpha = alph;

== matlab function simulation2_Fault/Current (North - East)/Current Rt ==
  data: u input; Rt output
function Rt = fcn(u)

R=[cos(u) -sin(u); sin(u) cos(u)];
Rt=transpose(R);

end

== matlab function simulation2_Fault/Thruster Dynamics/MATLAB Function ==
  data: alpha_actual input; thrust_actual input; actual_tau output; PosX input; PosY input
function actual_tau   = fcn(alpha_actual,thrust_actual,PosX,PosY)

    Alpha_surge =[cos(alpha_actual(1)) cos(alpha_actual(2)) cos(alpha_actual(3)) cos(alpha_actual(4)) cos(alpha_actual(5)) cos(alpha_actual(6))];  
    Alpha_sway = [sin(alpha_actual(1)) sin(alpha_actual(2)) sin(alpha_actual(3)) sin(alpha_actual(4)) sin(alpha_actual(5)) sin(alpha_actual(6))];
    Alpha_yaw = [sin(alpha_actual(1))*PosX(1)-cos(alpha_actual(1))*PosY(1) sin(alpha_actual(2))*PosX(2)-cos(alpha_actual(2))*PosY(2) ...
                 sin(alpha_actual(3))*PosX(3)-cos(alpha_actual(3))*PosY(3) sin(alpha_actual(4))*PosX(4)-cos(alpha_actual(4))*PosY(4) ...
                 sin(alpha_actual(5))*PosX(5)-cos(alpha_actual(5))*PosY(5) sin(alpha_actual(6))*PosX(6)-cos(alpha_actual(6))*PosY(6)];

    actual_tau = [Alpha_surge; Alpha_sway; Alpha_yaw]*thrust_actual;
end
